simulink model "car_speed_control_Student"  (R2026a)
settings: Solver=ode1  StopTime=20  FixedStep=0.01
values from neighbouring files (symbols this model uses):
  UT = legacy_plant_parameters(      vehicleParams,      simulationParams)    [run_open_loop_test.m]
undefined symbols (not defined in the file or in its folder): DiscIntNeverNeededParam, T_ADE, To_be_determined, v_ini
libraries: sl_discontinuities x1
(part 2 of 2)

== system car_speed_control_Student/Ego_Car_Model/PSG_first/Body Fixed Vehicle Dynamics/8dof_vehicle/4tyre_torque ==
  note: -20/Rw
  Tdf : Inport
  Tbfl : Inport  Port=2
  Tbfr : Inport  Port=3
  Tbrl : Inport  Port=4
  Tbrr : Inport  Port=5
  Fxfl : Inport  Port=6
  Fxfr : Inport  Port=7
  Fxrl : Inport  Port=8
  Fxrr : Inport  Port=9
  V_ini : Inport  Port=10
  Add2 : Sum  Inputs=--+
  Add3 : Sum  Inputs=+--
  Add4 : Sum  Inputs=--
  Add5 : Sum  Inputs=--
  Constant{,1..4} (5 alike) : Constant  Value=UT.Rw
  Discrete-Time Integrator{,1..3} (4 alike) : DiscreteIntegrator  InitialConditionSource=external  InitialCondition=UT.Veh_PSG_o(7)  SampleTime=UT.Ts_Veh  ICPrevOutput=DiscIntNeverNeededParam  ICPrevScaledInput=DiscIntNeverNeededParam
  Divide{,1..3} (4 alike) : Product  Inputs=*/
  Gain{1..3,5} (4 alike) : Gain  Gain=1/UT.Jw
  Product{,1..3} (4 alike) : Product
  Saturation{,1..3} (4 alike) : Saturate  UpperLimit=100/UT.Rw  LowerLimit=-20/UT.Rw
  omega_fl : Outport  VectorParamsAs1DForOutWhenUnconnected=off
  omega_fr : Outport  Port=2  VectorParamsAs1DForOutWhenUnconnected=off
  omega_rl : Outport  Port=3  VectorParamsAs1DForOutWhenUnconnected=off
  omega_rr : Outport  Port=4  VectorParamsAs1DForOutWhenUnconnected=off
  wires:
  Gain3/1 -> Discrete-Time Integrator3/1
  Product/1 -> Add2/1
  Tdf/1 -> Add3/1, Add2/3
  Constant/1 -> Product/2, Product3/1, Product2/1, Product1/1
  Product3/1 -> Add5/2
  Product2/1 -> Add4/2
  Tbfl/1 -> Add2/2
  Discrete-Time Integrator/1 -> Saturation/1
  Gain1/1 -> Discrete-Time Integrator1/1
  Discrete-Time Integrator1/1 -> Saturation1/1
  Gain2/1 -> Discrete-Time Integrator2/1
  Discrete-Time Integrator2/1 -> Saturation2/1
  Discrete-Time Integrator3/1 -> Saturation3/1
  Tbrl/1 -> Add4/1
  Add3/1 -> Gain1/1
  Add2/1 -> Gain5/1
  Add4/1 -> Gain2/1
  Add5/1 -> Gain3/1
  Gain5/1 -> Discrete-Time Integrator/1
  Fxfl/1 -> Product/1
  Fxfr/1 -> Product1/2
  Fxrl/1 -> Product2/2
  Fxrr/1 -> Product3/2
  Saturation/1 -> omega_fl/1
  Saturation1/1 -> omega_fr/1
  Saturation2/1 -> omega_rl/1
  Saturation3/1 -> omega_rr/1
  Product1/1 -> Add3/3
  Tbfr/1 -> Add3/2
  Tbrr/1 -> Add5/1
  Divide/1 -> Discrete-Time Integrator/2
  Constant1/1 -> Divide/2
  Constant2/1 -> Divide1/2
  Divide1/1 -> Discrete-Time Integrator1/2
  Divide2/1 -> Discrete-Time Integrator2/2
  Constant3/1 -> Divide2/2
  Constant4/1 -> Divide3/2
  Divide3/1 -> Discrete-Time Integrator3/2
  V_ini/1 -> Divide3/1, Divide2/1, Divide1/1, Divide/1

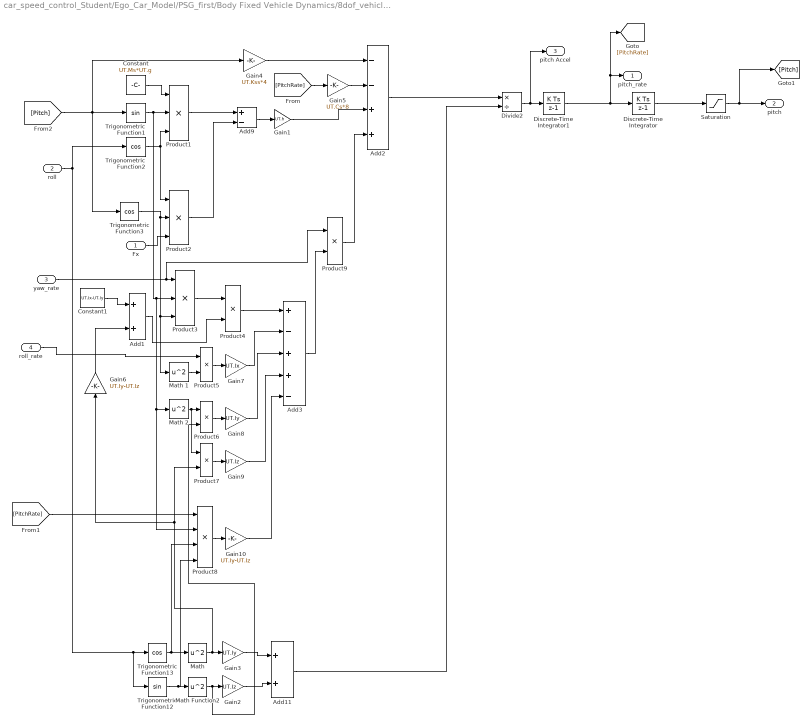
== system car_speed_control_Student/Ego_Car_Model/PSG_first/Body Fixed Vehicle Dynamics/8dof_vehicle/Pitch  ==
  Fx : Inport
  roll : Inport  Port=2
  yaw_rate : Inport  Port=3
  roll_rate : Inport  Port=4
  Add1 : Sum
  Add11 : Sum
  Add2 : Sum  Inputs=--++
  Add3 : Sum  Inputs=+-++-
  Add9 : Sum  Inputs=+-
  Constant : Constant  Value=UT.Ms*UT.g
  Constant1 : Constant  Value=UT.Ix-UT.Iy
  Discrete-Time Integrator : DiscreteIntegrator  SampleTime=UT.Ts_Veh  ICPrevOutput=DiscIntNeverNeededParam  ICPrevScaledInput=DiscIntNeverNeededParam
  Discrete-Time Integrator1 : DiscreteIntegrator  SampleTime=UT.Ts_Veh  ICPrevOutput=DiscIntNeverNeededParam  ICPrevScaledInput=DiscIntNeverNeededParam
  Divide2 : Product  Inputs=*/
  Gain1 : Gain  Gain=UT.h
  Gain10 : Gain  Gain=UT.Iy-UT.Iz
  Gain2 : Gain  Gain=UT.Iz
  Gain3 : Gain  Gain=UT.Iy
  Gain4 : Gain  Gain=UT.Kss*4
  Gain5 : Gain  Gain=UT.Cs*8
  Gain6 : Gain  Gain=UT.Iy-UT.Iz
  Gain7 : Gain  Gain=UT.Ix
  Gain8 : Gain  Gain=UT.Iy
  Gain9 : Gain  Gain=UT.Iz
  "Math " : Math  Operator=square  SignedPower=on
  Math 1 : Math  Operator=square  SignedPower=on
  Math 2 : Math  Operator=square  SignedPower=on
  Math Function2 : Math  Operator=square  SignedPower=on
  Product1 : Product  Inputs=3
  Product2 : Product  Inputs=3
  Product3 : Product  Inputs=3
  Product{4..7,9} (5 alike) : Product
  Product8 : Product  Inputs=4
  Saturation : Saturate  UpperLimit=0.18  LowerLimit=-0.18
  Trigonometric Function1 : Trigonometry
  Trigonometric Function12 : Trigonometry
  Trigonometric Function13 : Trigonometry  Operator=cos
  Trigonometric Function2 : Trigonometry  Operator=cos
  Trigonometric Function3 : Trigonometry  Operator=cos
  pitch_rate : Outport  VectorParamsAs1DForOutWhenUnconnected=off
  pitch : Outport  Port=2  VectorParamsAs1DForOutWhenUnconnected=off
  pitch Accel : Outport  Port=3  VectorParamsAs1DForOutWhenUnconnected=off
  wires:
  Discrete-Time Integrator/1 -> Saturation/1
  Add2/1 -> Divide2/1
  Product9/1 -> Add2/4
  Add3/1 -> Product9/2
  Gain10/1 -> Add3/5
  [PitchRate] -> Product8/1
  Product8/1 -> Gain10/1
  Gain9/1 -> Add3/4
  Product7/1 -> Gain9/1
  Math Function2/1 -> Gain2/1, Product6/2
  Gain8/1 -> Add3/3
  Trigonometric Function1/1 -> Product3/2, Math 2/1, Product8/2, Product1/2
  Math 2/1 -> Product6/1, Product7/1
  Product6/1 -> Gain8/1
  Gain7/1 -> Add3/2
  Product5/1 -> Gain7/1
  Math 1/1 -> Product5/2
  roll_rate/1 -> Product5/1
  Product4/1 -> Add3/1
  Add1/1 -> Product4/2
  Gain6/1 -> Add1/2
  Constant1/1 -> Add1/1
  Product3/1 -> Product4/1
  yaw_rate/1 -> Product3/1, Product9/1
  [PitchRate] -> Gain5/1
  Divide2/1 -> Discrete-Time Integrator1/1, pitch Accel/1
  Gain5/1 -> Add2/2
  Gain4/1 -> Add2/1
  Gain1/1 -> Add2/3
  Product2/1 -> Add9/2
  Trigonometric Function3/1 -> Product2/2, Product3/3, Math 1/1
  Fx/1 -> Product2/3
  Product1/1 -> Add9/1
  Trigonometric Function2/1 -> Product2/1, Product1/3
  Constant/1 -> Product1/1
  [Pitch] -> Trigonometric Function1/1, Trigonometric Function3/1, Gain4/1
  Add11/1 -> Divide2/2
  Gain2/1 -> Add11/2
  Trigonometric Function12/1 -> Math Function2/1, Product8/4
  Gain3/1 -> Add11/1
  "Math "/1 -> Gain3/1, Gain6/1, Product7/2
  Trigonometric Function13/1 -> "Math "/1, Product8/3
  Add9/1 -> Gain1/1
  roll/1 -> Trigonometric Function2/1, Trigonometric Function13/1, Trigonometric Function12/1
  Discrete-Time Integrator1/1 -> Discrete-Time Integrator/1, pitch_rate/1, [PitchRate]
  Saturation/1 -> pitch/1, [Pitch]

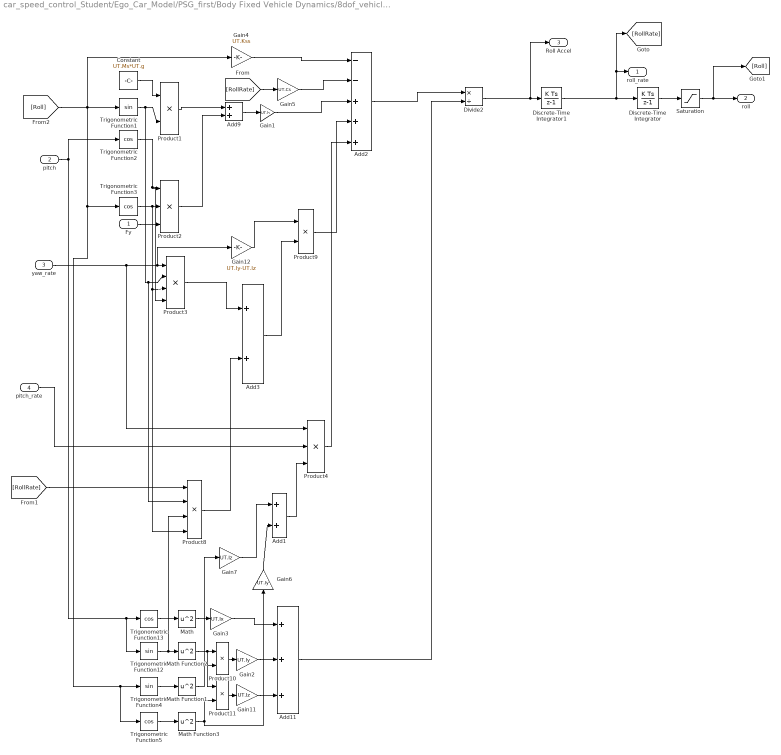
== system car_speed_control_Student/Ego_Car_Model/PSG_first/Body Fixed Vehicle Dynamics/8dof_vehicle/Roll ==
  Fy : Inport
  pitch : Inport  Port=2
  yaw_rate : Inport  Port=3
  pitch_rate : Inport  Port=4
  Add1 : Sum
  Add11 : Sum  Inputs=+++
  Add2 : Sum  Inputs=--+++
  Add3 : Sum
  Add9 : Sum
  Constant : Constant  Value=UT.Ms*UT.g
  Discrete-Time Integrator : DiscreteIntegrator  SampleTime=UT.Ts_Veh  ICPrevOutput=DiscIntNeverNeededParam  ICPrevScaledInput=DiscIntNeverNeededParam
  Discrete-Time Integrator1 : DiscreteIntegrator  SampleTime=UT.Ts_Veh  ICPrevOutput=DiscIntNeverNeededParam  ICPrevScaledInput=DiscIntNeverNeededParam
  Divide2 : Product  Inputs=*/
  Gain1 : Gain  Gain=UT.h
  Gain11 : Gain  Gain=UT.Iz
  Gain12 : Gain  Gain=UT.Iy-UT.Iz
  Gain2 : Gain  Gain=UT.Iy
  Gain3 : Gain  Gain=UT.Ix
  Gain4 : Gain  Gain=UT.Kss
  Gain5 : Gain  Gain=UT.Cs
  Gain6 : Gain  Gain=UT.Iy
  Gain7 : Gain  Gain=UT.Iz
  "Math " : Math  Operator=square  SignedPower=on
  Math Function1 : Math  Operator=square  SignedPower=on
  Math Function2 : Math  Operator=square  SignedPower=on
  Math Function3 : Math  Operator=square  SignedPower=on
  Product{1,9..11} (4 alike) : Product
  Product2 : Product  Inputs=3
  Product3 : Product  Inputs=4
  Product4 : Product  Inputs=3
  Product8 : Product  Inputs=4
  Saturation : Saturate  UpperLimit=45  LowerLimit=-45
  Trigonometric Function1 : Trigonometry
  Trigonometric Function12 : Trigonometry
  Trigonometric Function{2..3,5,13} (4 alike) : Trigonometry  Operator=cos
  Trigonometric Function4 : Trigonometry
  roll_rate : Outport  VectorParamsAs1DForOutWhenUnconnected=off
  roll : Outport  Port=2  VectorParamsAs1DForOutWhenUnconnected=off
  Roll Accel : Outport  Port=3  VectorParamsAs1DForOutWhenUnconnected=off
  wires:
  Discrete-Time Integrator1/1 -> [RollRate], roll_rate/1, Discrete-Time Integrator/1
  Divide2/1 -> Discrete-Time Integrator1/1, Roll Accel/1
  Product4/1 -> Add2/5
  Add1/1 -> Product4/3
  Gain7/1 -> Add1/1
  Gain6/1 -> Add1/2
  pitch_rate/1 -> Product4/2
  Gain12/1 -> Product9/1
  Math Function3/1 -> Gain6/1, Product11/2
  Trigonometric Function5/1 -> Math Function3/1
  Product11/1 -> Gain11/1
  Gain11/1 -> Add11/3
  Gain2/1 -> Add11/2
  Math Function1/1 -> Product10/2, Gain7/1
  Trigonometric Function4/1 -> Math Function1/1
  Product10/1 -> Gain2/1
  Saturation/1 -> [Roll], roll/1
  Discrete-Time Integrator/1 -> Saturation/1
  pitch/1 -> Trigonometric Function12/1, Trigonometric Function13/1, Trigonometric Function2/1
  Add9/1 -> Gain1/1
  Trigonometric Function13/1 -> "Math "/1
  "Math "/1 -> Gain3/1
  Gain3/1 -> Add11/1
  Trigonometric Function12/1 -> Math Function2/1, Product8/3
  Add11/1 -> Divide2/2
  [Roll] -> Gain4/1, Trigonometric Function3/1, Trigonometric Function4/1, Trigonometric Function5/1, Trigonometric Function1/1
  Constant/1 -> Product1/1
  Trigonometric Function2/1 -> Product2/1, Product3/4
  Product1/1 -> Add9/1
  Fy/1 -> Product2/3
  Trigonometric Function3/1 -> Product3/3, Product8/4, Product2/2
  Product2/1 -> Add9/2
  Gain1/1 -> Add2/3
  Gain4/1 -> Add2/1
  Gain5/1 -> Add2/2
  [RollRate] -> Gain5/1
  yaw_rate/1 -> Gain12/1, Product3/1, Product4/1
  Product3/1 -> Add3/1
  Trigonometric Function1/1 -> Product1/2, Product8/2, Product3/2
  Math Function2/1 -> Product10/1, Product11/1
  Product8/1 -> Add3/2
  [RollRate] -> Product8/1
  Add3/1 -> Product9/2
  Product9/1 -> Add2/4
  Add2/1 -> Divide2/1

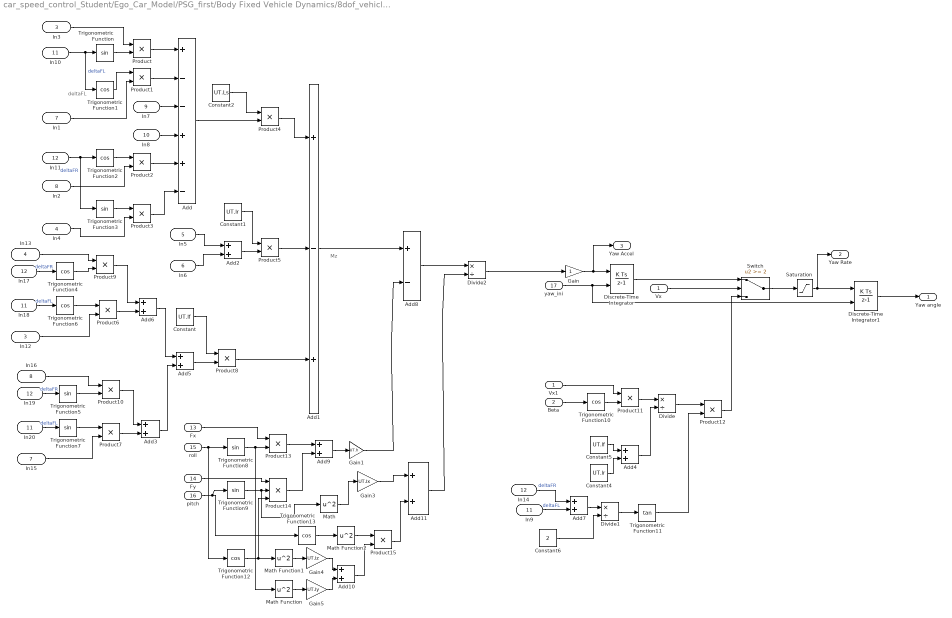
== system car_speed_control_Student/Ego_Car_Model/PSG_first/Body Fixed Vehicle Dynamics/8dof_vehicle/Yaw Dynamics ==
  note: deltaFL
  note: Mz
  Vx : Inport
  Beta : Inport  Port=2
  In3 : Inport  Port=3
  In4 : Inport  Port=4
  In5 : Inport  Port=5
  In6 : Inport  Port=6
  In1 : Inport  Port=7
  In2 : Inport  Port=8
  In7 : Inport  Port=9
  In8 : Inport  Port=10
  In10 : Inport  Port=11
  In11 : Inport  Port=12
  Fx : Inport  Port=13
  Fy : Inport  Port=14
  roll : Inport  Port=15
  "pitch " : Inport  Port=16
  yaw_ini : Inport  Port=17
  Add : Sum  Inputs=+--++-
  Add1 : Sum  Inputs=+-+
  Add{2..7,9..11} (9 alike) : Sum
  Add8 : Sum  Inputs=+-
  Constant : Constant  Value=UT.lf
  Constant1 : Constant  Value=UT.lr
  Constant2 : Constant  Value=UT.Ls
  Constant4 : Constant  Value=UT.lr
  Constant5 : Constant  Value=UT.lf
  Constant6 : Constant  Value=2
  Discrete-Time Integrator : DiscreteIntegrator  InitialConditionSource=external  InitialCondition=UT.Veh_PSG_o(3)  SampleTime=UT.Ts_Veh  ICPrevOutput=DiscIntNeverNeededParam  ICPrevScaledInput=DiscIntNeverNeededParam
  Discrete-Time Integrator1 : DiscreteIntegrator  InitialConditionSource=external  InitialCondition=UT.Veh_PSG_o(3)  SampleTime=UT.Ts_Veh  ICPrevOutput=DiscIntNeverNeededParam  ICPrevScaledInput=DiscIntNeverNeededParam
  Divide : Product  Inputs=*/
  Divide1 : Product  Inputs=*/
  Divide2 : Product  Inputs=*/
  Gain : Gain
  Gain1 : Gain  Gain=UT.h
  Gain3 : Gain  Gain=UT.Ix
  Gain4 : Gain  Gain=UT.Iz
  Gain5 : Gain  Gain=UT.Iy
  In12 : InportShadow  Port=3
  In13 : InportShadow  Port=4
  In14 : InportShadow  Port=12
  In15 : InportShadow  Port=7
  In16 : InportShadow  Port=8
  In17 : InportShadow  Port=12
  In18 : InportShadow  Port=11
  In19 : InportShadow  Port=12
  In20 : InportShadow  Port=11
  In9 : InportShadow  Port=11
  "Math " : Math  Operator=square  SignedPower=on
  Math Function : Math  Operator=square  SignedPower=on
  Math Function1 : Math  Operator=square  SignedPower=on
  Math Function2 : Math  Operator=square  SignedPower=on
  Product{,1..13,15} (15 alike) : Product
  Product14 : Product  Inputs=3
  Saturation : Saturate  UpperLimit=50*3.14/180  LowerLimit=-50*3.14/180  SampleTime=UT.Ts_Veh
  Switch : Switch  Threshold=2  SaturateOnIntegerOverflow=off  InputSameDT=off
  Trigonometric Function{,3,5,7..9} (6 alike) : Trigonometry
  Trigonometric Function{1..2,4,6,10,12..13} (7 alike) : Trigonometry  Operator=cos
  Trigonometric Function11 : Trigonometry  Operator=tan
  Vx1 : InportShadow
  Yaw angle : Outport  VectorParamsAs1DForOutWhenUnconnected=off
  Yaw Rate : Outport  Port=2  VectorParamsAs1DForOutWhenUnconnected=off
  Yaw Accel : Outport  Port=3  VectorParamsAs1DForOutWhenUnconnected=off
  wires:
  Divide2/1 -> Gain/1
  Add11/1 -> Divide2/2
  "Math "/1 -> Gain3/1
  Gain3/1 -> Add11/1
  Product15/1 -> Add11/2
  Math Function2/1 -> Product15/1
  Trigonometric Function13/1 -> Math Function2/1
  Add10/1 -> Product15/2
  Gain4/1 -> Add10/1
  Math Function1/1 -> Gain4/1
  Gain5/1 -> Add10/2
  Math Function/1 -> Gain5/1
  Add8/1 -> Divide2/1
  Gain1/1 -> Add8/2
  Add9/1 -> Gain1/1
  Product14/1 -> Add9/2
  Trigonometric Function12/1 -> Math Function1/1, Product14/3
  Trigonometric Function9/1 -> Product14/2, "Math "/1
  "pitch "/1 -> Trigonometric Function13/1, Trigonometric Function9/1
  Fy/1 -> Product14/1
  Product13/1 -> Add9/1
  Fx/1 -> Product13/1
  Trigonometric Function8/1 -> Product13/2, Math Function/1
  roll/1 -> Trigonometric Function12/1, Trigonometric Function8/1
  In14/1 -> Add7/1  "deltaFR"
  In9/1 -> Add7/2  "deltaFL"
  In20/1 -> Trigonometric Function7/1  "deltaFL"
  In19/1 -> Trigonometric Function5/1  "deltaFR"
  Trigonometric Function7/1 -> Product7/1
  Trigonometric Function5/1 -> Product10/2
  Product7/1 -> Add3/2
  Product10/1 -> Add3/1
  In15/1 -> Product7/2
  Add3/1 -> Add5/2
  In16/1 -> Product10/1
  In17/1 -> Trigonometric Function4/1  "deltaFR"
  In18/1 -> Trigonometric Function6/1  "deltaFL"
  Trigonometric Function6/1 -> Product6/1
  Trigonometric Function4/1 -> Product9/2
  Product6/1 -> Add6/2
  Product9/1 -> Add6/1
  In12/1 -> Product6/2
  In11/1 -> Trigonometric Function2/1, Trigonometric Function3/1  "deltaFR"
  Product8/1 -> Add1/3
  Constant/1 -> Product8/1
  Add5/1 -> Product8/2
  Add6/1 -> Add5/1
  Add1/1 -> Add8/1
  In13/1 -> Product9/1
  Product5/1 -> Add1/2
  Constant1/1 -> Product5/1
  Add2/1 -> Product5/2
  In6/1 -> Add2/2
  In5/1 -> Add2/1
  Product4/1 -> Add1/1
  Constant2/1 -> Product4/1
  Add/1 -> Product4/2
  Product3/1 -> Add/6
  In4/1 -> Product3/2
  Trigonometric Function3/1 -> Product3/1
  Product2/1 -> Add/5
  In2/1 -> Product2/2
  Trigonometric Function2/1 -> Product2/1
  In8/1 -> Add/4
  In7/1 -> Add/3
  Product1/1 -> Add/2
  In1/1 -> Product1/2
  Trigonometric Function1/1 -> Product1/1
  Product/1 -> Add/1
  Trigonometric Function/1 -> Product/2
  In3/1 -> Product/1
  In10/1 -> Trigonometric Function/1, Trigonometric Function1/1  "deltaFL"
  Saturation/1 -> Yaw Rate/1, Discrete-Time Integrator1/1
  Product12/1 -> Switch/3
  Switch/1 -> Saturation/1
  Divide/1 -> Product12/1
  Trigonometric Function11/1 -> Product12/2
  Divide1/1 -> Trigonometric Function11/1
  Product11/1 -> Divide/1
  Trigonometric Function10/1 -> Product11/2
  Vx1/1 -> Product11/1
  Beta/1 -> Trigonometric Function10/1
  Constant6/1 -> Divide1/2
  Add7/1 -> Divide1/1
  Add4/1 -> Divide/2
  Constant5/1 -> Add4/1
  Constant4/1 -> Add4/2
  Vx/1 -> Switch/2
  Gain/1 -> Discrete-Time Integrator/1, Yaw Accel/1
  Discrete-Time Integrator1/1 -> Yaw angle/1
  Discrete-Time Integrator/1 -> Switch/1
  yaw_ini/1 -> Discrete-Time Integrator/2, Discrete-Time Integrator1/2

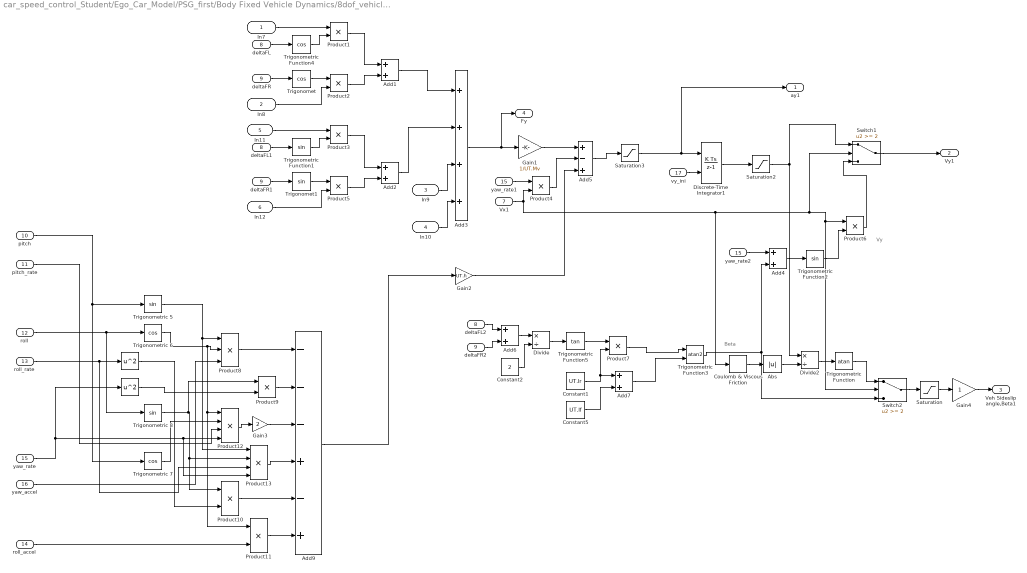
== system car_speed_control_Student/Ego_Car_Model/PSG_first/Body Fixed Vehicle Dynamics/8dof_vehicle/lateral ==
  note: Vy
  note: Beta
  In7 : Inport
  In8 : Inport  Port=2
  In9 : Inport  Port=3
  In10 : Inport  Port=4
  In11 : Inport  Port=5
  In12 : Inport  Port=6
  Vx1 : Inport  Port=7
  deltaFL : Inport  Port=8
  deltaFR : Inport  Port=9
  pitch : Inport  Port=10
  pitch_rate : Inport  Port=11
  roll : Inport  Port=12
  roll_rate : Inport  Port=13
  roll_accel : Inport  Port=14
  yaw_rate : Inport  Port=15
  yaw_accel : Inport  Port=16
  vy_ini : Inport  Port=17
  " " : Math  Operator=square  SignedPower=on
  " " : Math  Operator=square  SignedPower=on
  Abs : Abs  SaturateOnIntegerOverflow=off
  Add{1..2,4,6..7} (5 alike) : Sum
  Add3 : Sum  Inputs=++++
  Add5 : Sum  Inputs=+-+
  Add9 : Sum  Inputs=---+-+
  Constant1 : Constant  Value=UT.lr
  Constant2 : Constant  Value=2
  Constant5 : Constant  Value=UT.lf
  Coulomb & Viscous Friction : sl_discontinuities/Coulomb & Viscous Friction  offset=0.01  gain=1
  Discrete-Time Integrator1 : DiscreteIntegrator  InitialConditionSource=external  InitialCondition=UT.Veh_PSG_o(2)  SampleTime=UT.Ts_Veh  ICPrevOutput=DiscIntNeverNeededParam  ICPrevScaledInput=DiscIntNeverNeededParam
  Divide : Product  Inputs=*/
  Divide2 : Product  Inputs=*/
  Gain1 : Gain  Gain=1/UT.Mv
  Gain2 : Gain  Gain=UT.h
  Gain3 : Gain  Gain=2
  Gain4 : Gain
  Product{1..3,5..7,9..11} (9 alike) : Product
  Product12 : Product  Inputs=4
  Product13 : Product  Inputs=4
  Product4 : Product  RndMeth=Zero
  Product8 : Product  Inputs=3
  Saturation : Saturate  UpperLimit=10*3.14/180  LowerLimit=-10*3.14/180
  Saturation2 : Saturate  UpperLimit=100  LowerLimit=-100
  Saturation3 : Saturate  UpperLimit=6  LowerLimit=-6
  Switch1 : Switch  Threshold=2  SaturateOnIntegerOverflow=off  InputSameDT=off
  Switch2 : Switch  Threshold=2  SaturateOnIntegerOverflow=off  InputSameDT=off
  Trigonomet : Trigonometry  Operator=cos
  Trigonomet1 : Trigonometry
  Trigonometric 5 : Trigonometry
  Trigonometric 6 : Trigonometry  Operator=cos
  Trigonometric 7 : Trigonometry  Operator=cos
  Trigonometric 8 : Trigonometry
  Trigonometric Function : Trigonometry  Operator=atan
  Trigonometric Function1 : Trigonometry
  Trigonometric Function2 : Trigonometry
  Trigonometric Function3 : Trigonometry  Operator=atan2
  Trigonometric Function4 : Trigonometry  Operator=cos
  Trigonometric Function5 : Trigonometry  Operator=tan
  deltaFL1 : InportShadow  Port=8
  deltaFL2 : InportShadow  Port=8
  deltaFR1 : InportShadow  Port=9
  deltaFR2 : InportShadow  Port=9
  yaw_rate1 : InportShadow  Port=15
  yaw_rate2 : InportShadow  Port=15
  ay1 : Outport  VectorParamsAs1DForOutWhenUnconnected=off
  Vy1 : Outport  Port=2  VectorParamsAs1DForOutWhenUnconnected=off
  Veh Sideslip angle,Beta1 : Outport  Port=3  VectorParamsAs1DForOutWhenUnconnected=off
  Fy : Outport  Port=4  VectorParamsAs1DForOutWhenUnconnected=off
  wires:
  Coulomb & Viscous Friction/1 -> Abs/1
  Switch1/1 -> Vy1/1
  Saturation3/1 -> ay1/1, Discrete-Time Integrator1/1
  Gain4/1 -> Veh Sideslip angle,Beta1/1
  Add9/1 -> Gain2/1
  Add3/1 -> Gain1/1, Fy/1
  Trigonometric Function/1 -> Switch2/1
  roll_accel/1 -> Product11/2
  " "/1 -> Product10/2
  " "/1 -> Product9/2
  Product11/1 -> Add9/6
  Trigonometric 8/1 -> Product10/1, Product13/2, Product9/1
  Product10/1 -> Add9/5
  Product13/1 -> Add9/4
  Trigonometric 7/1 -> Product12/2
  Gain3/1 -> Add9/3
  Product12/1 -> Gain3/1
  Product9/1 -> Add9/2
  Product8/1 -> Add9/1
  Trigonometric 5/1 -> Product8/1, Product13/1
  Trigonometric 6/1 -> Product8/2, Product12/1, Product11/1
  roll/1 -> Trigonometric 6/1, Trigonometric 8/1
  pitch/1 -> Trigonometric 5/1, Trigonometric 7/1
  yaw_accel/1 -> Product8/3
  yaw_rate/1 -> " "/1, Product12/4, Product13/4
  roll_rate/1 -> " "/1, Product13/3
  pitch_rate/1 -> Product12/3
  Gain2/1 -> Add5/3
  Saturation/1 -> Gain4/1
  Switch2/1 -> Saturation/1
  Add7/1 -> Trigonometric Function3/2
  Abs/1 -> Divide2/2
  Vx1/1 -> Switch1/2, Switch2/2, Product6/1, Coulomb & Viscous Friction/1, Product4/2
  Trigonometric Function3/1 -> Switch2/3, Add4/2
  Divide2/1 -> Trigonometric Function/1
  Product6/1 -> Switch1/3
  Saturation2/1 -> Switch1/1, Divide2/1
  Constant5/1 -> Add7/2
  Product7/1 -> Trigonometric Function3/1
  Constant1/1 -> Add7/1, Product7/2
  Trigonometric Function5/1 -> Product7/1
  Divide/1 -> Trigonometric Function5/1
  Constant2/1 -> Divide/2
  Add6/1 -> Divide/1
  deltaFR2/1 -> Add6/2
  deltaFL2/1 -> Add6/1
  Trigonometric Function2/1 -> Product6/2
  Add4/1 -> Trigonometric Function2/1
  yaw_rate2/1 -> Add4/1
  deltaFR1/1 -> Trigonomet1/1
  deltaFL1/1 -> Trigonometric Function1/1
  Add2/1 -> Add3/2
  Product5/1 -> Add2/2
  Product3/1 -> Add2/1
  Trigonometric Function1/1 -> Product3/2
  Trigonomet1/1 -> Product5/1
  In12/1 -> Product5/2
  In11/1 -> Product3/1
  Product2/1 -> Add1/2
  Product1/1 -> Add1/1
  deltaFR/1 -> Trigonomet/1
  deltaFL/1 -> Trigonometric Function4/1
  Trigonometric Function4/1 -> Product1/2
  Trigonomet/1 -> Product2/1
  Discrete-Time Integrator1/1 -> Saturation2/1
  Product4/1 -> Add5/2
  In10/1 -> Add3/4
  In9/1 -> Add3/3
  Add1/1 -> Add3/1
  yaw_rate1/1 -> Product4/1
  In8/1 -> Product2/2
  In7/1 -> Product1/1
  Add5/1 -> Saturation3/1
  Gain1/1 -> Add5/1
  vy_ini/1 -> Discrete-Time Integrator1/2

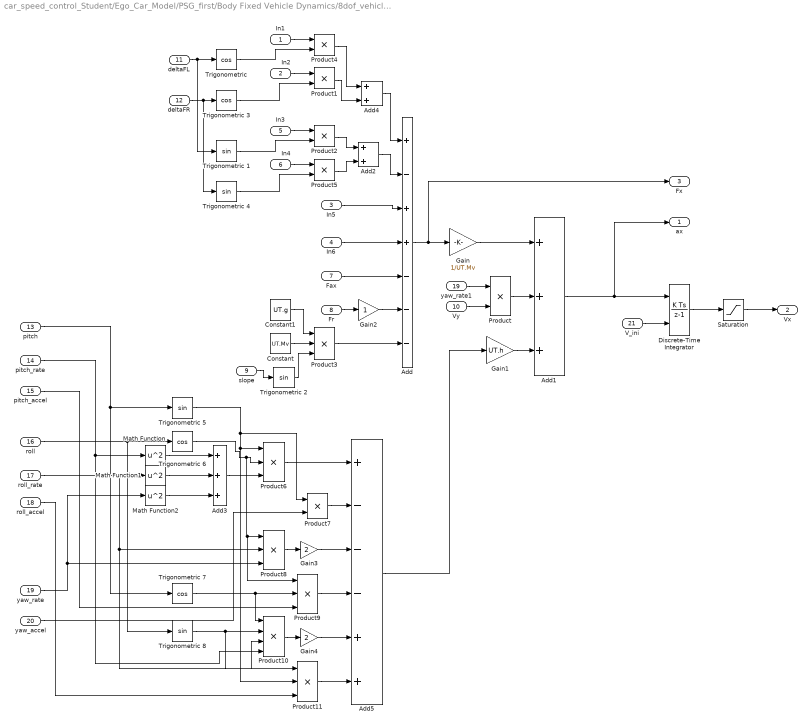
== system car_speed_control_Student/Ego_Car_Model/PSG_first/Body Fixed Vehicle Dynamics/8dof_vehicle/longitudinal ==
  In1 : Inport
  In2 : Inport  Port=2
  In5 : Inport  Port=3
  In6 : Inport  Port=4
  In3 : Inport  Port=5
  In4 : Inport  Port=6
  Fax : Inport  Port=7
  Fr : Inport  Port=8
  slope : Inport  Port=9
  Vy : Inport  Port=10
  deltaFL : Inport  Port=11
  deltaFR : Inport  Port=12
  pitch : Inport  Port=13
  pitch_rate : Inport  Port=14
  pitch_accel : Inport  Port=15
  roll : Inport  Port=16
  roll_rate : Inport  Port=17
  roll_accel : Inport  Port=18
  yaw_rate : Inport  Port=19
  yaw_accel : Inport  Port=20
  V_ini : Inport  Port=21
  Add : Sum  Inputs=+-++---
  Add1 : Sum  Inputs=+++
  Add2 : Sum
  Add3 : Sum  Inputs=+++
  Add4 : Sum
  Add5 : Sum  Inputs=+---++
  Constant : Constant  Value=UT.Mv
  Constant1 : Constant  Value=UT.g
  Discrete-Time Integrator : DiscreteIntegrator  InitialConditionSource=external  InitialCondition=UT.Veh_PSG_o(1)  SampleTime=UT.Ts_Veh  ICPrevOutput=DiscIntNeverNeededParam  ICPrevScaledInput=DiscIntNeverNeededParam
  Gain : Gain  Gain=1/UT.Mv
  Gain1 : Gain  Gain=UT.h
  Gain2 : Gain
  Gain3 : Gain  Gain=2
  Gain4 : Gain  Gain=2
  Math Function : Math  Operator=square  SignedPower=on
  Math Function1 : Math  Operator=square  SignedPower=on
  Math Function2 : Math  Operator=square  SignedPower=on
  Product{,1..2,4..5,7} (6 alike) : Product
  Product10 : Product  Inputs=4
  Product{3,6,8..9,11} (5 alike) : Product  Inputs=3
  Saturation : Saturate  UpperLimit=50  LowerLimit=0
  Trigonometric {,3,6..7} (4 alike) : Trigonometry  Operator=cos
  Trigonometric {1..2,4..5,8} (5 alike) : Trigonometry
  yaw_rate1 : InportShadow  Port=19
  ax : Outport  VectorParamsAs1DForOutWhenUnconnected=off
  Vx : Outport  Port=2  VectorParamsAs1DForOutWhenUnconnected=off
  Fx : Outport  Port=3  VectorParamsAs1DForOutWhenUnconnected=off
  wires:
  Add5/1 -> Gain1/1
  roll_accel/1 -> Product11/3
  Product11/1 -> Add5/6
  Trigonometric 8/1 -> Product10/2, Product11/1
  Product10/1 -> Gain4/1
  Gain4/1 -> Add5/5
  Product9/1 -> Add5/4
  pitch_accel/1 -> Product9/3
  Trigonometric 7/1 -> Product9/2, Product10/1
  Gain3/1 -> Add5/3
  Product8/1 -> Gain3/1
  Product7/1 -> Add5/2
  yaw_accel/1 -> Product7/2
  Product6/1 -> Add5/1
  Trigonometric 5/1 -> Product6/1, Product11/2, Product7/1
  Trigonometric 6/1 -> Product6/2, Product8/1, Product9/1
  roll/1 -> Trigonometric 6/1, Trigonometric 8/1
  pitch/1 -> Trigonometric 5/1, Trigonometric 7/1
  Add3/1 -> Product6/3
  Math Function2/1 -> Add3/3
  Math Function1/1 -> Add3/2
  Math Function/1 -> Add3/1
  yaw_rate/1 -> Math Function2/1, Product8/3
  roll_rate/1 -> Math Function1/1, Product8/2, Product10/3
  pitch_rate/1 -> Math Function/1, Product10/4
  Gain1/1 -> Add1/3
  Saturation/1 -> Vx/1
  Product5/1 -> Add2/2
  Product2/1 -> Add2/1
  Trigonometric 4/1 -> Product5/2
  Trigonometric 1/1 -> Product2/2
  Trigonometric 3/1 -> Product1/2
  deltaFR/1 -> Trigonometric 3/1, Trigonometric 4/1
  "Trigonometric "/1 -> Product4/2
  deltaFL/1 -> "Trigonometric "/1, Trigonometric 1/1
  In2/1 -> Product1/1
  Product1/1 -> Add4/2
  Gain2/1 -> Add/6
  Constant/1 -> Product3/2
  Constant1/1 -> Product3/1
  Trigonometric 2/1 -> Product3/3
  Add1/1 -> ax/1, Discrete-Time Integrator/1
  In6/1 -> Add/4
  In5/1 -> Add/3
  Add2/1 -> Add/2
  In4/1 -> Product5/1
  In3/1 -> Product2/1
  Add4/1 -> Add/1
  Product4/1 -> Add4/1
  In1/1 -> Product4/1
  Gain/1 -> Add1/1
  Product/1 -> Add1/2
  Add/1 -> Gain/1, Fx/1
  Vy/1 -> Product/2
  yaw_rate1/1 -> Product/1
  Product3/1 -> Add/7
  slope/1 -> Trigonometric 2/1
  Fr/1 -> Gain2/1
  Fax/1 -> Add/5
  Discrete-Time Integrator/1 -> Saturation/1
  V_ini/1 -> Discrete-Time Integrator/2

== system car_speed_control_Student/Ego_Car_Model/PSG_first/Body Fixed Vehicle Dynamics/Driving Resistance Subsystem/Aerodynamic Resistance ==
  note: increaesd to 0.75*...
  note: Vx=m/s
  note: Fa=0.5*p*Cd*A(Vx+Vw)^2
  Vx : Inport
  X Aerodynamic Fcn : Fcn  Expr=0.75*UT.rho*UT.Cd*UT.Awind*(u(1)+UT.Vw)^2  SampleTime=UT.Ts_Veh
  Fa : Outport  VectorParamsAs1DForOutWhenUnconnected=off
  wires:
  Vx/1 -> X Aerodynamic Fcn/1
  X Aerodynamic Fcn/1 -> Fa/1

== system car_speed_control_Student/Ego_Car_Model/PSG_first/Body Fixed Vehicle Dynamics/Driving Resistance Subsystem/Rolling resistance ==
  note: added *2
  Vx : Inport
  Rolling resistance Fcn1 : Fcn  Expr=(0.005+(1/2.013)*(0.01+0.0095*((3.6*u(1))/100)^2))*UT.Mv*UT.g*2  SampleTime=UT.Ts_Veh
  Fr : Outport  VectorParamsAs1DForOutWhenUnconnected=off
  wires:
  Rolling resistance Fcn1/1 -> Fr/1
  Vx/1 -> Rolling resistance Fcn1/1

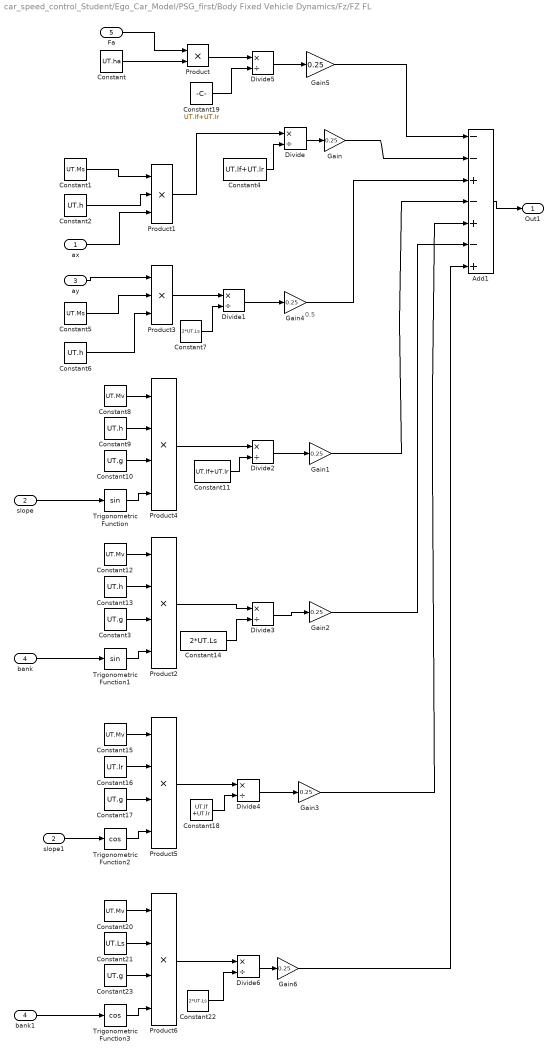
== system car_speed_control_Student/Ego_Car_Model/PSG_first/Body Fixed Vehicle Dynamics/Fz/FZ FL ==
  note: 0.5
  ax : Inport
  slope : Inport  Port=2
  ay : Inport  Port=3
  bank : Inport  Port=4
  Fa : Inport  Port=5
  Add1 : Sum  Inputs=--+-+-+
  Constant : Constant  Value=UT.ha
  Constant1 : Constant  Value=UT.Ms
  Constant{3,10,17,23} (4 alike) : Constant  Value=UT.g
  Constant11 : Constant  Value=UT.lf+UT.lr
  Constant{8,12,15,20} (4 alike) : Constant  Value=UT.Mv
  Constant{2,6,9,13} (4 alike) : Constant  Value=UT.h
  Constant14 : Constant  Value=2*UT.Ls
  Constant16 : Constant  Value=UT.lr
  Constant18 : Constant  Value=UT.lf +UT.lr
  Constant19 : Constant  Value=UT.lf+UT.lr
  Constant21 : Constant  Value=UT.Ls
  Constant22 : Constant  Value=2*UT.Ls
  Constant4 : Constant  Value=UT.lf+UT.lr
  Constant5 : Constant  Value=UT.Ms
  Constant7 : Constant  Value=2*UT.Ls
  Divide{,1..6} (7 alike) : Product  Inputs=*/
  Gain{,1..6} (7 alike) : Gain  Gain=0.25
  Product : Product
  Product1 : Product  Inputs=3
  Product{2,4..6} (4 alike) : Product  Inputs=4
  Product3 : Product  Inputs=3
  Trigonometric Function : Trigonometry
  Trigonometric Function1 : Trigonometry
  Trigonometric Function2 : Trigonometry  Operator=cos
  Trigonometric Function3 : Trigonometry  Operator=cos
  bank1 : InportShadow  Port=4
  slope1 : InportShadow  Port=2
  Out1 : Outport  VectorParamsAs1DForOutWhenUnconnected=off
  wires:
  Gain6/1 -> Add1/7
  Divide6/1 -> Gain6/1
  Constant22/1 -> Divide6/2
  Product6/1 -> Divide6/1
  Trigonometric Function3/1 -> Product6/4
  bank1/1 -> Trigonometric Function3/1
  Constant23/1 -> Product6/3
  Constant21/1 -> Product6/2
  Constant20/1 -> Product6/1
  Gain2/1 -> Add1/6
  Gain4/1 -> Add1/3
  Gain3/1 -> Add1/5
  Gain1/1 -> Add1/4
  Gain/1 -> Add1/2
  Gain5/1 -> Add1/1
  Divide5/1 -> Gain5/1
  Constant19/1 -> Divide5/2
  Product/1 -> Divide5/1
  Constant/1 -> Product/2
  Fa/1 -> Product/1
  Product1/1 -> Divide/1
  Add1/1 -> Out1/1
  Divide4/1 -> Gain3/1
  Product5/1 -> Divide4/1
  Constant18/1 -> Divide4/2
  slope1/1 -> Trigonometric Function2/1
  Trigonometric Function2/1 -> Product5/4
  Constant17/1 -> Product5/3
  Constant16/1 -> Product5/2
  Constant15/1 -> Product5/1
  Divide3/1 -> Gain2/1
  Constant14/1 -> Divide3/2
  Product2/1 -> Divide3/1
  Trigonometric Function1/1 -> Product2/4
  bank/1 -> Trigonometric Function1/1
  Constant3/1 -> Product2/3
  Constant13/1 -> Product2/2
  Constant12/1 -> Product2/1
  Product4/1 -> Divide2/1
  Divide2/1 -> Gain1/1
  Constant11/1 -> Divide2/2
  Trigonometric Function/1 -> Product4/4
  slope/1 -> Trigonometric Function/1
  Constant10/1 -> Product4/3
  Constant9/1 -> Product4/2
  Constant8/1 -> Product4/1
  Divide1/1 -> Gain4/1
  Divide/1 -> Gain/1
  Constant7/1 -> Divide1/2
  Product3/1 -> Divide1/1
  Constant6/1 -> Product3/3
  Constant5/1 -> Product3/2
  ay/1 -> Product3/1
  Constant4/1 -> Divide/2
  ax/1 -> Product1/3
  Constant2/1 -> Product1/2
  Constant1/1 -> Product1/1

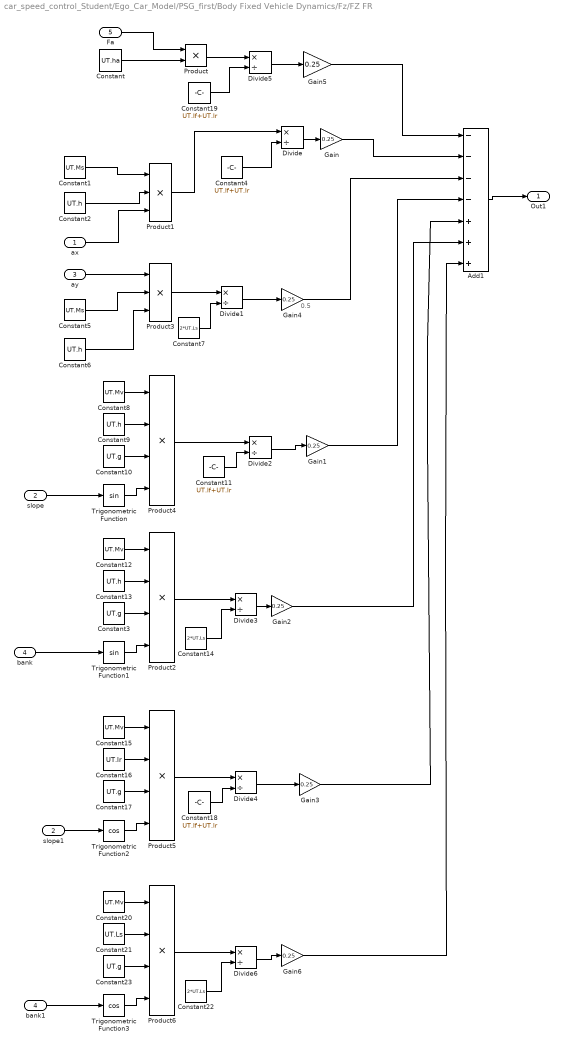
== system car_speed_control_Student/Ego_Car_Model/PSG_first/Body Fixed Vehicle Dynamics/Fz/FZ FR ==
  note: 0.5
  ax : Inport
  slope : Inport  Port=2
  ay : Inport  Port=3
  bank : Inport  Port=4
  Fa : Inport  Port=5
  Add1 : Sum  Inputs=----+++
  Constant : Constant  Value=UT.ha
  Constant1 : Constant  Value=UT.Ms
  Constant{3,10,17,23} (4 alike) : Constant  Value=UT.g
  Constant{4,11,18..19} (4 alike) : Constant  Value=UT.lf+UT.lr
  Constant{8,12,15,20} (4 alike) : Constant  Value=UT.Mv
  Constant{2,6,9,13} (4 alike) : Constant  Value=UT.h
  Constant14 : Constant  Value=2*UT.Ls
  Constant16 : Constant  Value=UT.lr
  Constant21 : Constant  Value=UT.Ls
  Constant22 : Constant  Value=2*UT.Ls
  Constant5 : Constant  Value=UT.Ms
  Constant7 : Constant  Value=2*UT.Ls
  Divide{,1..6} (7 alike) : Product  Inputs=*/
  Gain{,1..6} (7 alike) : Gain  Gain=0.25
  Product : Product
  Product1 : Product  Inputs=3
  Product{2,4..6} (4 alike) : Product  Inputs=4
  Product3 : Product  Inputs=3
  Trigonometric Function : Trigonometry
  Trigonometric Function1 : Trigonometry
  Trigonometric Function2 : Trigonometry  Operator=cos
  Trigonometric Function3 : Trigonometry  Operator=cos
  bank1 : InportShadow  Port=4
  slope1 : InportShadow  Port=2
  Out1 : Outport  VectorParamsAs1DForOutWhenUnconnected=off
  wires:
  Constant1/1 -> Product1/1
  Constant2/1 -> Product1/2
  ax/1 -> Product1/3
  Constant4/1 -> Divide/2
  ay/1 -> Product3/1
  Constant5/1 -> Product3/2
  Constant6/1 -> Product3/3
  Product3/1 -> Divide1/1
  Constant7/1 -> Divide1/2
  Divide/1 -> Gain/1
  Divide1/1 -> Gain4/1
  Constant8/1 -> Product4/1
  Constant9/1 -> Product4/2
  Constant10/1 -> Product4/3
  slope/1 -> Trigonometric Function/1
  Trigonometric Function/1 -> Product4/4
  Constant11/1 -> Divide2/2
  Divide2/1 -> Gain1/1
  Product4/1 -> Divide2/1
  Constant12/1 -> Product2/1
  Constant13/1 -> Product2/2
  Constant3/1 -> Product2/3
  bank/1 -> Trigonometric Function1/1
  Trigonometric Function1/1 -> Product2/4
  Product2/1 -> Divide3/1
  Constant14/1 -> Divide3/2
  Divide3/1 -> Gain2/1
  Constant15/1 -> Product5/1
  Constant16/1 -> Product5/2
  Constant17/1 -> Product5/3
  Trigonometric Function2/1 -> Product5/4
  slope1/1 -> Trigonometric Function2/1
  Constant18/1 -> Divide4/2
  Product5/1 -> Divide4/1
  Divide4/1 -> Gain3/1
  Add1/1 -> Out1/1
  Product1/1 -> Divide/1
  Fa/1 -> Product/1
  Constant/1 -> Product/2
  Product/1 -> Divide5/1
  Constant19/1 -> Divide5/2
  Divide5/1 -> Gain5/1
  Gain5/1 -> Add1/1
  Gain/1 -> Add1/2
  Gain1/1 -> Add1/4
  Gain3/1 -> Add1/5
  Gain4/1 -> Add1/3
  Gain2/1 -> Add1/6
  Constant20/1 -> Product6/1
  Constant21/1 -> Product6/2
  Constant23/1 -> Product6/3
  bank1/1 -> Trigonometric Function3/1
  Trigonometric Function3/1 -> Product6/4
  Product6/1 -> Divide6/1
  Constant22/1 -> Divide6/2
  Divide6/1 -> Gain6/1
  Gain6/1 -> Add1/7

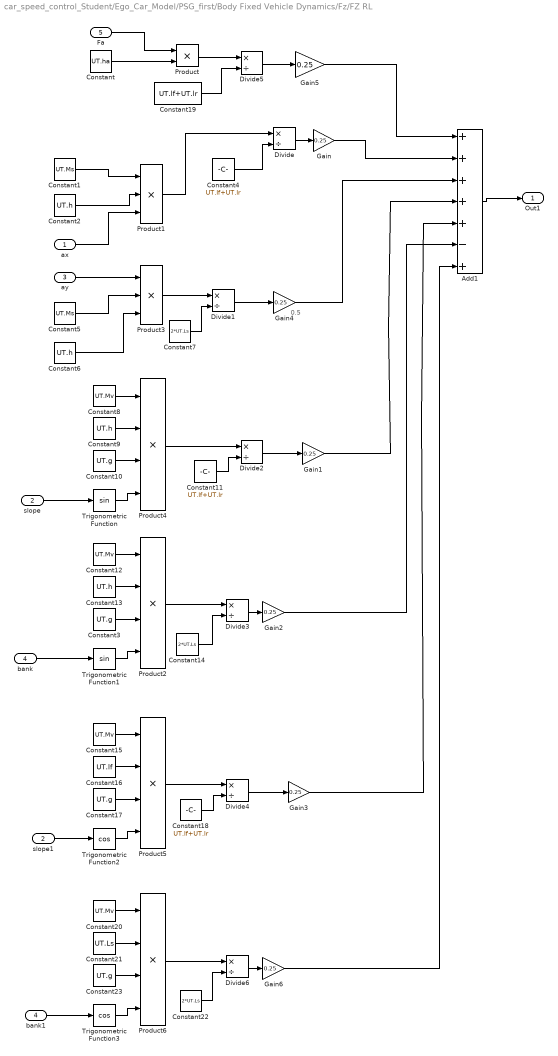
== system car_speed_control_Student/Ego_Car_Model/PSG_first/Body Fixed Vehicle Dynamics/Fz/FZ RL ==
  note: 0.5
  ax : Inport
  slope : Inport  Port=2
  ay : Inport  Port=3
  bank : Inport  Port=4
  Fa : Inport  Port=5
  Add1 : Sum  Inputs=+++++-+
  Constant : Constant  Value=UT.ha
  Constant1 : Constant  Value=UT.Ms
  Constant{3,10,17,23} (4 alike) : Constant  Value=UT.g
  Constant{4,11,18..19} (4 alike) : Constant  Value=UT.lf+UT.lr
  Constant{8,12,15,20} (4 alike) : Constant  Value=UT.Mv
  Constant{2,6,9,13} (4 alike) : Constant  Value=UT.h
  Constant14 : Constant  Value=2*UT.Ls
  Constant16 : Constant  Value=UT.lf
  Constant21 : Constant  Value=UT.Ls
  Constant22 : Constant  Value=2*UT.Ls
  Constant5 : Constant  Value=UT.Ms
  Constant7 : Constant  Value=2*UT.Ls
  Divide{,1..6} (7 alike) : Product  Inputs=*/
  Gain{,1..6} (7 alike) : Gain  Gain=0.25
  Product : Product
  Product1 : Product  Inputs=3
  Product{2,4..6} (4 alike) : Product  Inputs=4
  Product3 : Product  Inputs=3
  Trigonometric Function : Trigonometry
  Trigonometric Function1 : Trigonometry
  Trigonometric Function2 : Trigonometry  Operator=cos
  Trigonometric Function3 : Trigonometry  Operator=cos
  bank1 : InportShadow  Port=4
  slope1 : InportShadow  Port=2
  Out1 : Outport  VectorParamsAs1DForOutWhenUnconnected=off
  wires:
  Constant1/1 -> Product1/1
  Constant2/1 -> Product1/2
  ax/1 -> Product1/3
  Constant4/1 -> Divide/2
  ay/1 -> Product3/1
  Constant5/1 -> Product3/2
  Constant6/1 -> Product3/3
  Product3/1 -> Divide1/1
  Constant7/1 -> Divide1/2
  Divide/1 -> Gain/1
  Divide1/1 -> Gain4/1
  Constant8/1 -> Product4/1
  Constant9/1 -> Product4/2
  Constant10/1 -> Product4/3
  slope/1 -> Trigonometric Function/1
  Trigonometric Function/1 -> Product4/4
  Constant11/1 -> Divide2/2
  Divide2/1 -> Gain1/1
  Product4/1 -> Divide2/1
  Constant12/1 -> Product2/1
  Constant13/1 -> Product2/2
  Constant3/1 -> Product2/3
  bank/1 -> Trigonometric Function1/1
  Trigonometric Function1/1 -> Product2/4
  Product2/1 -> Divide3/1
  Constant14/1 -> Divide3/2
  Divide3/1 -> Gain2/1
  Constant15/1 -> Product5/1
  Constant16/1 -> Product5/2
  Constant17/1 -> Product5/3
  Trigonometric Function2/1 -> Product5/4
  slope1/1 -> Trigonometric Function2/1
  Constant18/1 -> Divide4/2
  Product5/1 -> Divide4/1
  Divide4/1 -> Gain3/1
  Add1/1 -> Out1/1
  Product1/1 -> Divide/1
  Fa/1 -> Product/1
  Constant/1 -> Product/2
  Product/1 -> Divide5/1
  Constant19/1 -> Divide5/2
  Divide5/1 -> Gain5/1
  Gain5/1 -> Add1/1
  Gain/1 -> Add1/2
  Gain1/1 -> Add1/4
  Gain3/1 -> Add1/5
  Gain4/1 -> Add1/3
  Gain2/1 -> Add1/6
  Constant20/1 -> Product6/1
  Constant21/1 -> Product6/2
  Constant23/1 -> Product6/3
  bank1/1 -> Trigonometric Function3/1
  Trigonometric Function3/1 -> Product6/4
  Product6/1 -> Divide6/1
  Constant22/1 -> Divide6/2
  Divide6/1 -> Gain6/1
  Gain6/1 -> Add1/7

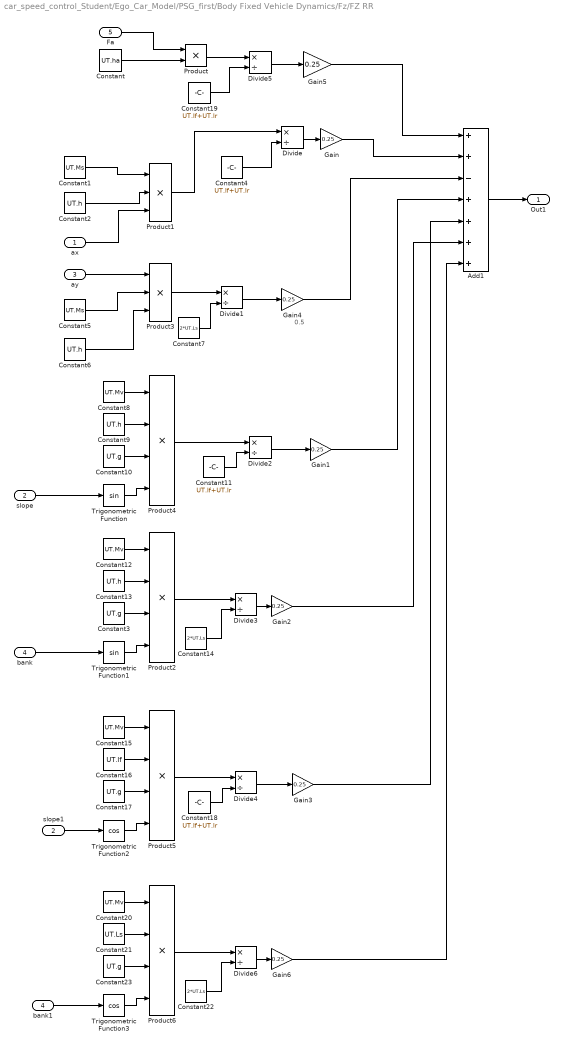
== system car_speed_control_Student/Ego_Car_Model/PSG_first/Body Fixed Vehicle Dynamics/Fz/FZ RR ==
  note: 0.5
  ax : Inport
  slope : Inport  Port=2
  ay : Inport  Port=3
  bank : Inport  Port=4
  Fa : Inport  Port=5
  Add1 : Sum  Inputs=++-++++
  Constant : Constant  Value=UT.ha
  Constant1 : Constant  Value=UT.Ms
  Constant{3,10,17,23} (4 alike) : Constant  Value=UT.g
  Constant{4,11,18..19} (4 alike) : Constant  Value=UT.lf+UT.lr
  Constant{8,12,15,20} (4 alike) : Constant  Value=UT.Mv
  Constant{2,6,9,13} (4 alike) : Constant  Value=UT.h
  Constant14 : Constant  Value=2*UT.Ls
  Constant16 : Constant  Value=UT.lf
  Constant21 : Constant  Value=UT.Ls
  Constant22 : Constant  Value=2*UT.Ls
  Constant5 : Constant  Value=UT.Ms
  Constant7 : Constant  Value=2*UT.Ls
  Divide{,1..6} (7 alike) : Product  Inputs=*/
  Gain{,1..6} (7 alike) : Gain  Gain=0.25
  Product : Product
  Product1 : Product  Inputs=3
  Product{2,4..6} (4 alike) : Product  Inputs=4
  Product3 : Product  Inputs=3
  Trigonometric Function : Trigonometry
  Trigonometric Function1 : Trigonometry
  Trigonometric Function2 : Trigonometry  Operator=cos
  Trigonometric Function3 : Trigonometry  Operator=cos
  bank1 : InportShadow  Port=4
  slope1 : InportShadow  Port=2
  Out1 : Outport  VectorParamsAs1DForOutWhenUnconnected=off
  wires:
  Gain6/1 -> Add1/7
  Divide6/1 -> Gain6/1
  Constant22/1 -> Divide6/2
  Product6/1 -> Divide6/1
  Trigonometric Function3/1 -> Product6/4
  bank1/1 -> Trigonometric Function3/1
  Constant23/1 -> Product6/3
  Constant21/1 -> Product6/2
  Constant20/1 -> Product6/1
  Gain2/1 -> Add1/6
  Gain4/1 -> Add1/3
  Gain3/1 -> Add1/5
  Gain1/1 -> Add1/4
  Gain/1 -> Add1/2
  Gain5/1 -> Add1/1
  Divide5/1 -> Gain5/1
  Constant19/1 -> Divide5/2
  Product/1 -> Divide5/1
  Constant/1 -> Product/2
  Fa/1 -> Product/1
  Product1/1 -> Divide/1
  Add1/1 -> Out1/1
  Divide4/1 -> Gain3/1
  Product5/1 -> Divide4/1
  Constant18/1 -> Divide4/2
  slope1/1 -> Trigonometric Function2/1
  Trigonometric Function2/1 -> Product5/4
  Constant17/1 -> Product5/3
  Constant16/1 -> Product5/2
  Constant15/1 -> Product5/1
  Divide3/1 -> Gain2/1
  Constant14/1 -> Divide3/2
  Product2/1 -> Divide3/1
  Trigonometric Function1/1 -> Product2/4
  bank/1 -> Trigonometric Function1/1
  Constant3/1 -> Product2/3
  Constant13/1 -> Product2/2
  Constant12/1 -> Product2/1
  Product4/1 -> Divide2/1
  Divide2/1 -> Gain1/1
  Constant11/1 -> Divide2/2
  Trigonometric Function/1 -> Product4/4
  slope/1 -> Trigonometric Function/1
  Constant10/1 -> Product4/3
  Constant9/1 -> Product4/2
  Constant8/1 -> Product4/1
  Divide1/1 -> Gain4/1
  Divide/1 -> Gain/1
  Constant7/1 -> Divide1/2
  Product3/1 -> Divide1/1
  Constant6/1 -> Product3/3
  Constant5/1 -> Product3/2
  ay/1 -> Product3/1
  Constant4/1 -> Divide/2
  ax/1 -> Product1/3
  Constant2/1 -> Product1/2
  Constant1/1 -> Product1/1

== matlab function car_speed_control_Student/Algebraic Derivative Estimator/MATLAB Function ==
  data: U input; Dot_U output; Ts input; u_init input
function Dot_U = buffer(U, Ts, u_init)
    N =12; % Sliding window length
    persistent y;
    if isempty(y)
        y=u_init*ones(N+1,1); % We initialized a sliding window here
    end

    y = [U;y(1:end-1)];
    T = Ts*N;
    P = zeros(1,N+1);
    P_alpha = P;
    for k = 1:N+1
        tao_k = (k-1)*Ts;
        P(k) = ; % to be filled 
        if((k==1)||(k==N+1))
            P_alpha(k) = P(k)*Ts/2;
        else
            P_alpha(k) = P(k)*Ts;
        end
    end
    
    Dot_U = ; % to be filled

end

== matlab function car_speed_control_Student/MFC/Torque_constraint (N.m.) ==
  data: Torque_unconstraint input; Torque_considering_constraint output; T_real_last input; T_max input; deltaT_max input
function Torque_considering_constraint = f(Torque_unconstraint, T_real_last, T_max, deltaT_max)
  % To be filled
end
